simulink model "f"  (R2024a)
settings: Solver=VariableStepAuto  StartTime=0.0  StopTime=5  RelTol=1e-3
model workspace (MAT data in the model file):
  frequency_needed = 1
libraries: spsIGBTDiodeLib x6, spsAsynchronousMachineSIUnitsLib x1, spsControlledVoltageSourceLib x1, dspstat3 x1, spsTriangleGeneratorLib x1, spsVoltageMeasurementLib x1, sps_lib x1
settings Model: Creator=jishankurane  LastModifiedBy=jishankurane

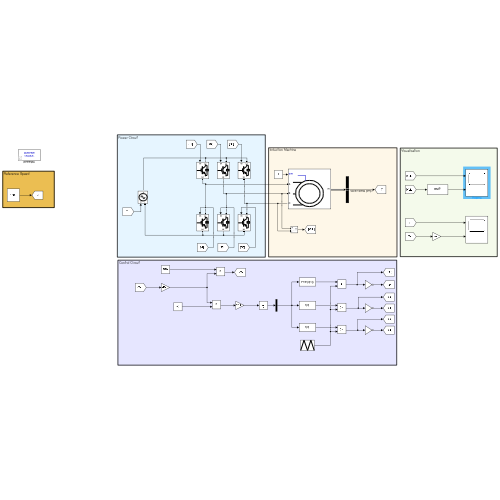
[thumbnail: Simulink's stored preview of the top-level diagram]
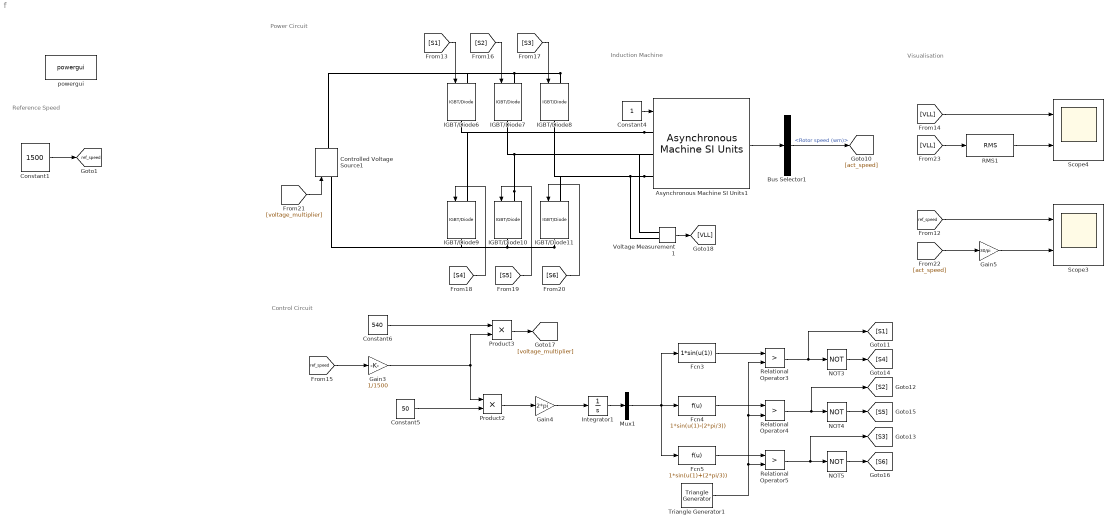
== system f ==
  note: Reference Speed
  note: Induction Machine
  note: Control Circuit
  note: Power Circuit
  note: Visualisation
  Asynchronous Machine SI Units1 : spsAsynchronousMachineSIUnitsLib/Asynchronous Machine SI Units  RotorType=Squirrel-cage  PresetModel=No  MechanicalLoad=Torque Tm  ShowDetailedParameters=on  ReferenceFrame=Rotor  Units=SI  MeasurementBus=off  NominalParameters=[1.845e+04 400 50]  VoltageRatio=1  Stator=[0.5968 0.0003495]  Rotor=[0.6258 0.005473]  Cage1=[0.4155 0.002066]  Cage2=[0.4168 0.0003495]  Lm=0.0354  Mechanical=[0.05 0.005879 2]  PolePairs=2  InitialConditions=[0 0 0 0 0 0 0 0]  SimulateSaturation=off  Saturation=[14.03593122, 27.81365428, 53.79336849, 72.68890987, 97.98006896, 148.6815601, 215.7428561, 302.9841135, 428.7778367 ; 230, 322, 414, 460, 506, 552, 598, 644, 690]  LoadFlowParameters=1492000  TsPowergui=0  TsBlock=-1  IterativeModel=Trapezoidal non iterative  IterativeDiscreteModel=Trapezoidal non iterative  Pmec=1.492e+006
  Bus Selector1 : BusSelector  OutputSignals=Mechanical.Rotor speed (wm)
  Constant1 : Constant  Value=1500
  Constant4 : Constant
  Constant5 : Constant  Value=50
  Constant6 : Constant  Value=540
  Controlled Voltage Source1 : spsControlledVoltageSourceLib/Controlled Voltage Source  Initialize=on  Source_Type=DC  Amplitude=540  Phase=0  Frequency=0  Measurements=None
  Fcn3 : Fcn  Expr=1*sin(u(1))
  Fcn4 : Fcn  Expr=1*sin(u(1)-(2*pi/3))
  Fcn5 : Fcn  Expr=1*sin(u(1)+(2*pi/3))
  Gain3 : Gain  Gain=1/1500
  Gain4 : Gain  Gain=2*pi
  Gain5 : Gain  Gain=30/pi
  IGBT/Diode{6..11} (6 alike) : spsIGBTDiodeLib/IGBT//Diode  Ron=1e-3  Rs=1e5  Cs=inf  Measurements=off
  Integrator1 : Integrator
  Mux1 : Mux  Inputs=1
  NOT3 : Logic  Operator=NOT  IconShape=distinctive  AllPortsSameDT=off  OutDataTypeStr=boolean
  NOT4 : Logic  Operator=NOT  IconShape=distinctive  AllPortsSameDT=off  OutDataTypeStr=boolean
  NOT5 : Logic  Operator=NOT  IconShape=distinctive  AllPortsSameDT=off  OutDataTypeStr=boolean
  Product2 : Product
  Product3 : Product
  RMS1 : dspstat3/RMS  run=off  directionMode=Each column  dimension=1  InputProcessing=Columns as channels (frame based)  reset_popup=None
  Relational Operator3 : RelationalOperator  Operator=>  OutDataTypeStr=boolean  RndMeth=Simplest  InputSameDT=off
  Relational Operator4 : RelationalOperator  Operator=>  OutDataTypeStr=boolean  RndMeth=Simplest  InputSameDT=off
  Relational Operator5 : RelationalOperator  Operator=>  OutDataTypeStr=boolean  RndMeth=Simplest  InputSameDT=off
  Scope3 : Scope  NumInputPorts=2
  Scope4 : Scope  NumInputPorts=2
  Triangle Generator1 : spsTriangleGeneratorLib/Triangle Generator  Freq=10e3  Phase=0  Ts=0
  Voltage Measurement1 : spsVoltageMeasurementLib/Voltage Measurement  PhasorSimulation=off  OutputType=Complex  PSBequivalent=0
  powergui : sps_lib/powergui  Priority=1  SimulationMode=Discrete  SampleTime=1e-5  frequency=60  Iterations=50  frequencyindice=50  Pbase=100e6  ErrMax=1e-4  UnitsV=kV  UnitsW=MW  buscounter=0  FunctionMessages=off  echomessages=off  EnableUseOfTLC=off  CurrentSourceSwitches=off  DisableSnubberDevices=off  DisableRonSwitches=off  DisableVfSwitches=off  DisplayEquations=off  AutomaticDiscreteSolvers=off  SolverType=Tustin/Backward Euler (TBE)  Interpol=off  ExternalGateDelay=off  methode=off  Ts=100  x0status=blocks  SPID=on  SwTol=0  HookPort=off  NonlinearTolerance=1e-4  nMaxIteration=100  ContinueOnMaxIteration=off  RestoreLinks=warning  ResistiveCurrentMeasurement=off  Frange=[0:2:500]  Ylog=off  Xlog=on  ShowGrid=off  save=off  variable=ZData  structure=0  ZoomFFT=off  StartTime=0.0  cycles=1  DisplayStyle=1  fundamental=60  FreqAxis=off  MaxFrequency=1000  frequencyindicesteady=1  RmsSteady=1  display=off
  tag scope: ref_speed=global
  wires:
  Constant1/1 -> [ref_speed]
  [voltage_multiplier] -> Controlled Voltage Source1/1
  Relational Operator5/1 -> [S3], NOT5/1
  Product2/1 -> Gain4/1
  [S4] -> IGBT/Diode9/1
  NOT5/1 -> [S6]
  Fcn4/1 -> Relational Operator4/1
  [VLL] -> Scope4/1
  Constant6/1 -> Product3/1
  [S6] -> IGBT/Diode11/1
  NOT4/1 -> [S5]
  Product3/1 -> [voltage_multiplier]
  [ref_speed] -> Gain3/1
  [act_speed] -> Gain5/1
  Bus Selector1/1 -> [act_speed]  "<Rotor speed (wm)>"
  Relational Operator3/1 -> [S1], NOT3/1
  Asynchronous Machine SI Units1/1 -> Bus Selector1/1
  Gain3/1 -> Product3/2, Product2/1
  Constant5/1 -> Product2/2
  Fcn3/1 -> Relational Operator3/1
  Triangle Generator1/1 -> Relational Operator3/2, Relational Operator4/2, Relational Operator5/2
  NOT3/1 -> [S4]
  [ref_speed] -> Scope3/1
  Voltage Measurement1/1 -> [VLL]
  [S5] -> IGBT/Diode10/1
  [S3] -> IGBT/Diode8/1
  [VLL] -> RMS1/1
  Constant4/1 -> Asynchronous Machine SI Units1/1
  RMS1/1 -> Scope4/2
  Relational Operator4/1 -> [S2], NOT4/1
  Gain5/1 -> Scope3/2
  [S2] -> IGBT/Diode7/1
  Integrator1/1 -> Mux1/1
  Mux1/1 -> Fcn4/1, Fcn3/1, Fcn5/1
  Fcn5/1 -> Relational Operator5/1
  [S1] -> IGBT/Diode6/1
  Gain4/1 -> Integrator1/1
  connections:
  Asynchronous Machine SI Units1/LConn3 -- Voltage Measurement1/LConn2 -- IGBT/Diode8/RConn1 -- IGBT/Diode11/LConn1
  IGBT/Diode11/RConn1 -- Controlled Voltage Source1/LConn1 -- IGBT/Diode9/RConn1 -- IGBT/Diode10/RConn1
  IGBT/Diode8/LConn1 -- IGBT/Diode7/LConn1 -- Controlled Voltage Source1/RConn1 -- IGBT/Diode6/LConn1
  IGBT/Diode10/LConn1 -- Asynchronous Machine SI Units1/LConn2 -- Voltage Measurement1/LConn1 -- IGBT/Diode7/RConn1
  Asynchronous Machine SI Units1/LConn1 -- IGBT/Diode6/RConn1 -- IGBT/Diode9/LConn1
